simulink model "ExampleStorageDoubleTempAssignment"  (R2016a)
settings: Solver=VariableStepAuto  StartTime=0.0  StopTime=3600*10  RelTol=1e-3
settings Model: Creator=chiavazzo  LastModifiedBy=chiavazzo

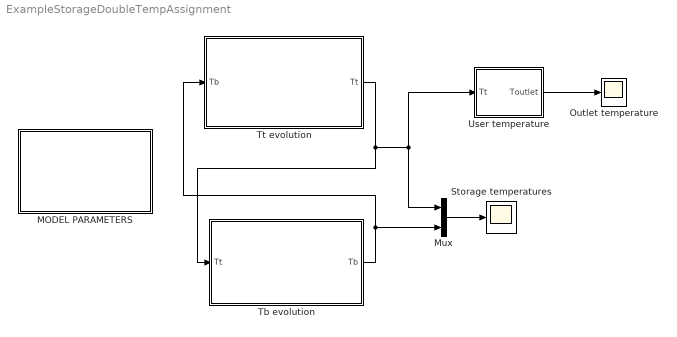
== system ExampleStorageDoubleTempAssignment ==
  " Outlet temperature" : Scope
  MODEL PARAMETERS : Subsystem
  Mux : Mux  Inputs=2
  Storage temperatures : Scope
  Tb evolution : Subsystem
  Tt evolution : Subsystem
  User temperature : Subsystem
  wires:
  Tt evolution/1(Tt) -> User temperature/1(Tt), Mux/1, Tb evolution/1(Tt)
  Tb evolution/1(Tb) -> Tt evolution/1(Tb), Mux/2
  Mux/1 -> Storage temperatures/1
  User temperature/1(Toutlet) -> " Outlet temperature"/1

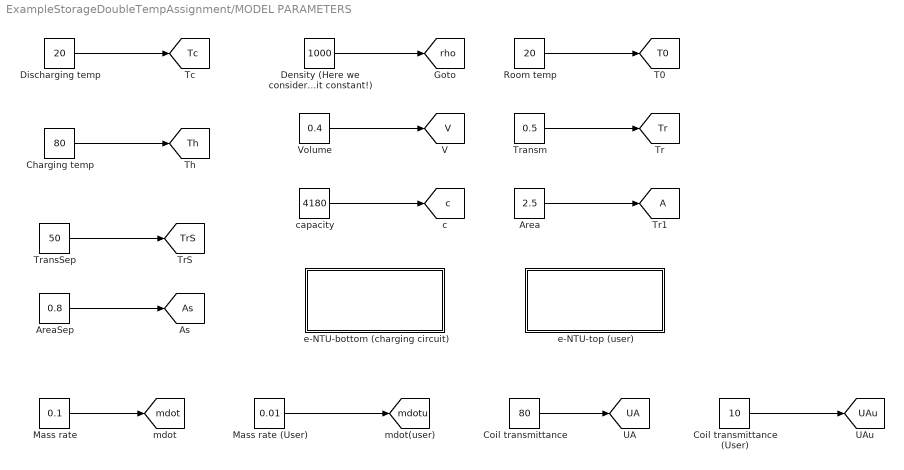
== system ExampleStorageDoubleTempAssignment/MODEL PARAMETERS ==
  Area : Constant  Value=2.5
  AreaSep : Constant  Value=0.8
  Charging temp : Constant  Value=80
  Coil transmittance : Constant  Value=80
  Coil transmittance (User) : Constant  Value=10
  Density (Here we consider it constant!) : Constant  Value=1000
  Discharging temp : Constant  Value=20
  Mass rate : Constant  Value=0.1
  Mass rate (User) : Constant  Value=0.01
  Room temp : Constant  Value=20
  TransSep : Constant  Value=50
  Transm : Constant  Value=0.5
  Volume : Constant  Value=0.4
  capacity : Constant  Value=4180
  e-NTU-bottom (charging circuit) : Subsystem
  e-NTU-top (user) : Subsystem
  tag scope: A=global, As=global, T0=global, Tc=global, Th=global, Tr=global, TrS=global, UA=global, UAu=global, V=global, c=global, mdot=global, mdotu=global, rho=global
  wires:
  Volume/1 -> [V]
  Coil transmittance/1 -> [UA]
  Mass rate/1 -> [mdot]
  capacity/1 -> [c]
  Area/1 -> [A]
  Room temp/1 -> [T0]
  Density (Here we consider it constant!)/1 -> [rho]
  Transm/1 -> [Tr]
  Charging temp/1 -> [Th]
  TransSep/1 -> [TrS]
  AreaSep/1 -> [As]
  Discharging temp/1 -> [Tc]
  Coil transmittance (User)/1 -> [UAu]
  Mass rate (User)/1 -> [mdotu]

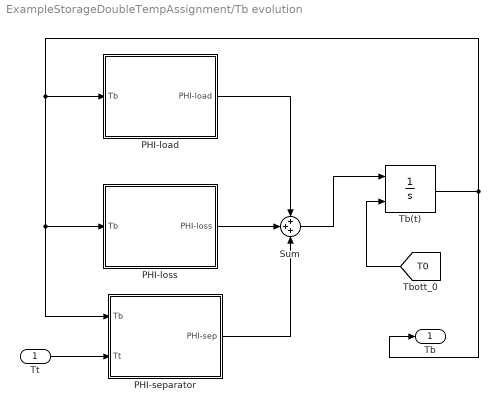
== system ExampleStorageDoubleTempAssignment/Tb evolution ==
  Tt : Inport
  PHI-load : Subsystem
  PHI-loss : Subsystem
  PHI-separator : Subsystem
  Sum : Sum  Inputs=+++
  Tb(t) : Integrator  InitialConditionSource=external
  Tb : Outport
  wires:
  PHI-loss/1(PHI-loss) -> Sum/2
  Sum/1 -> Tb(t)/1
  PHI-load/1(PHI-load) -> Sum/1
  [T0] -> Tb(t)/2
  Tb(t)/1 -> Tb/1, PHI-separator/1(Tb), PHI-loss/1(Tb), PHI-load/1(Tb)
  PHI-separator/1(PHI-sep) -> Sum/3
  Tt/1 -> PHI-separator/2(Tt)

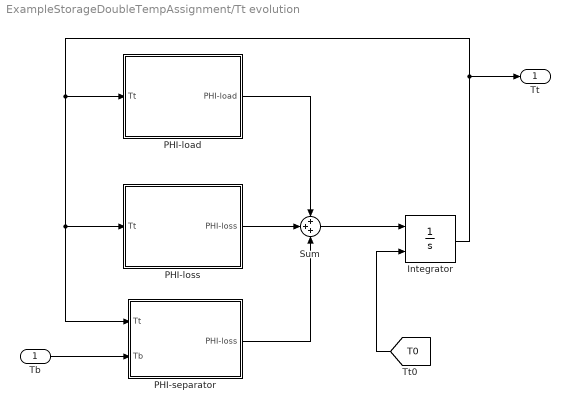
== system ExampleStorageDoubleTempAssignment/Tt evolution ==
  Tb : Inport
  Integrator : Integrator  InitialConditionSource=external
  PHI-load : Subsystem
  PHI-loss : Subsystem
  PHI-separator : Subsystem
  Sum : Sum  Inputs=+++
  Tt : Outport
  wires:
  PHI-loss/1(PHI-loss) -> Sum/2
  Sum/1 -> Integrator/1
  PHI-load/1(PHI-load) -> Sum/1
  [T0] -> Integrator/2
  Integrator/1 -> Tt/1, PHI-separator/1(Tt), PHI-loss/1(Tt), PHI-load/1(Tt)
  PHI-separator/1(PHI-loss) -> Sum/3
  Tb/1 -> PHI-separator/2(Tb)

== system ExampleStorageDoubleTempAssignment/User temperature ==
  Tt : Inport
  Product : Product
  Sum : Sum  Inputs=|+-
  Sum1 : Sum  Inputs=|++
  Toutlet : Outport
  wires:
  [epsu] -> Product/1
  Sum1/1 -> Toutlet/1
  Sum/1 -> Product/2
  [Tc] -> Sum/2
  [Tc] -> Sum1/1
  Product/1 -> Sum1/2
  Tt/1 -> Sum/1

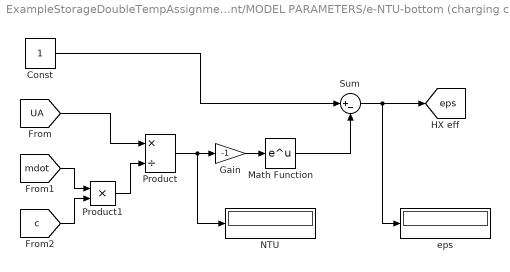
== system ExampleStorageDoubleTempAssignment/MODEL PARAMETERS/e-NTU-bottom (charging circuit) ==
  Const : Constant
  Gain : Gain  Gain=-1
  Math Function : Math  SaturateOnIntegerOverflow=on
  NTU : Display
  Product : Product  Inputs=*/
  Product1 : Product  Inputs=**
  Sum : Sum  Inputs=|+-
  eps : Display
  tag scope: eps=global
  wires:
  [mdot] -> Product1/1
  Product/1 -> NTU/1, Gain/1
  Product1/1 -> Product/2
  [UA] -> Product/1
  Sum/1 -> eps/1, [eps]
  Const/1 -> Sum/1
  Math Function/1 -> Sum/2
  Gain/1 -> Math Function/1
  [c] -> Product1/2

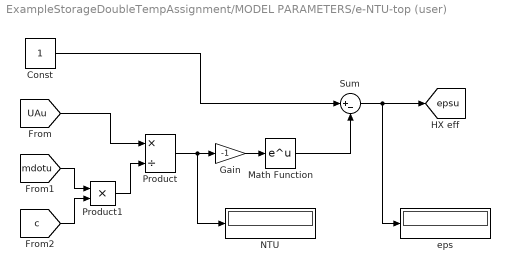
== system ExampleStorageDoubleTempAssignment/MODEL PARAMETERS/e-NTU-top (user) ==
  Const : Constant
  Gain : Gain  Gain=-1
  Math Function : Math  SaturateOnIntegerOverflow=on
  NTU : Display
  Product : Product  Inputs=*/
  Product1 : Product  Inputs=**
  Sum : Sum  Inputs=|+-
  eps : Display
  tag scope: epsu=global
  wires:
  [mdotu] -> Product1/1
  Product/1 -> NTU/1, Gain/1
  Product1/1 -> Product/2
  [UAu] -> Product/1
  Sum/1 -> eps/1, [epsu]
  Const/1 -> Sum/1
  Math Function/1 -> Sum/2
  Gain/1 -> Math Function/1
  [c] -> Product1/2

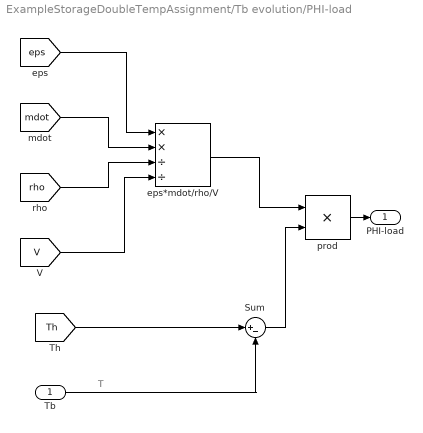
== system ExampleStorageDoubleTempAssignment/Tb evolution/PHI-load ==
  note: T
  Tb : Inport
  Sum : Sum  Inputs=|+-
  eps*mdot/rho/V : Product  Inputs=**//
  prod : Product  Inputs=**
  PHI-load : Outport
  wires:
  eps*mdot/rho/V/1 -> prod/1
  [V] -> eps*mdot/rho/V/4
  [mdot] -> eps*mdot/rho/V/2
  Sum/1 -> prod/2
  [rho] -> eps*mdot/rho/V/3
  [Th] -> Sum/1
  Tb/1 -> Sum/2
  prod/1 -> PHI-load/1
  [eps] -> eps*mdot/rho/V/1

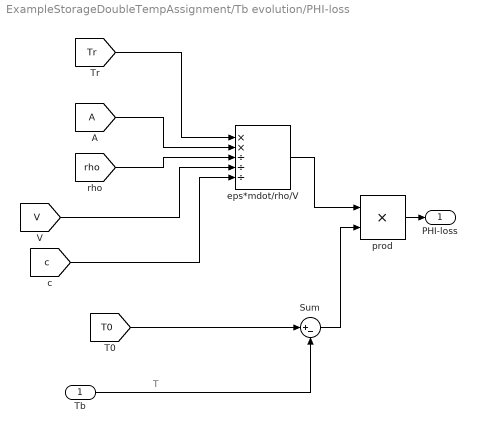
== system ExampleStorageDoubleTempAssignment/Tb evolution/PHI-loss ==
  note: T
  Tb : Inport
  Sum : Sum  Inputs=|+-
  eps*mdot/rho/V : Product  Inputs=**///
  prod : Product  Inputs=**
  PHI-loss : Outport
  wires:
  eps*mdot/rho/V/1 -> prod/1
  [V] -> eps*mdot/rho/V/4
  [A] -> eps*mdot/rho/V/2
  Sum/1 -> prod/2
  [rho] -> eps*mdot/rho/V/3
  [T0] -> Sum/1
  Tb/1 -> Sum/2
  prod/1 -> PHI-loss/1
  [Tr] -> eps*mdot/rho/V/1
  [c] -> eps*mdot/rho/V/5

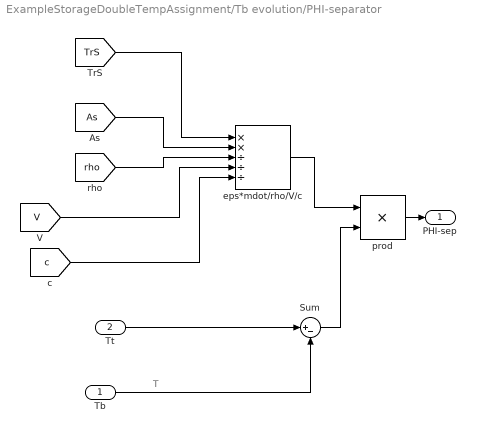
== system ExampleStorageDoubleTempAssignment/Tb evolution/PHI-separator ==
  note: T
  Tb : Inport
  Tt : Inport  Port=2
  Sum : Sum  Inputs=|+-
  eps*mdot/rho/V/c : Product  Inputs=**///
  prod : Product  Inputs=**
  PHI-sep : Outport
  wires:
  eps*mdot/rho/V/c/1 -> prod/1
  [V] -> eps*mdot/rho/V/c/4
  [As] -> eps*mdot/rho/V/c/2
  Sum/1 -> prod/2
  [rho] -> eps*mdot/rho/V/c/3
  Tt/1 -> Sum/1
  Tb/1 -> Sum/2
  prod/1 -> PHI-sep/1
  [TrS] -> eps*mdot/rho/V/c/1
  [c] -> eps*mdot/rho/V/c/5

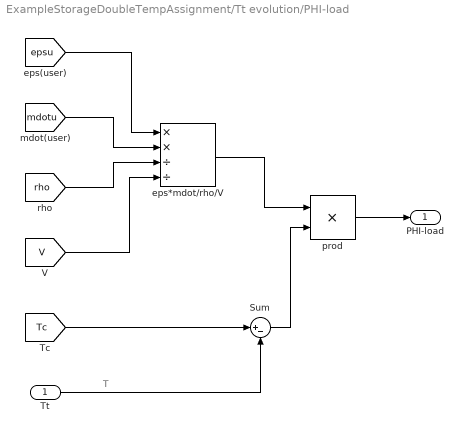
== system ExampleStorageDoubleTempAssignment/Tt evolution/PHI-load ==
  note: T
  Tt : Inport
  Sum : Sum  Inputs=|+-
  eps*mdot/rho/V : Product  Inputs=**//
  prod : Product  Inputs=**
  PHI-load : Outport
  wires:
  eps*mdot/rho/V/1 -> prod/1
  [V] -> eps*mdot/rho/V/4
  [mdotu] -> eps*mdot/rho/V/2
  Sum/1 -> prod/2
  [rho] -> eps*mdot/rho/V/3
  [Tc] -> Sum/1
  Tt/1 -> Sum/2
  prod/1 -> PHI-load/1
  [epsu] -> eps*mdot/rho/V/1

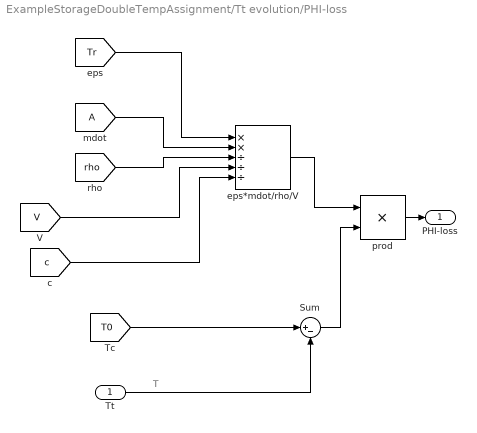
== system ExampleStorageDoubleTempAssignment/Tt evolution/PHI-loss ==
  note: T
  Tt : Inport
  Sum : Sum  Inputs=|+-
  eps*mdot/rho/V : Product  Inputs=**///
  prod : Product  Inputs=**
  PHI-loss : Outport
  wires:
  eps*mdot/rho/V/1 -> prod/1
  [V] -> eps*mdot/rho/V/4
  [A] -> eps*mdot/rho/V/2
  Sum/1 -> prod/2
  [rho] -> eps*mdot/rho/V/3
  [T0] -> Sum/1
  Tt/1 -> Sum/2
  prod/1 -> PHI-loss/1
  [Tr] -> eps*mdot/rho/V/1
  [c] -> eps*mdot/rho/V/5

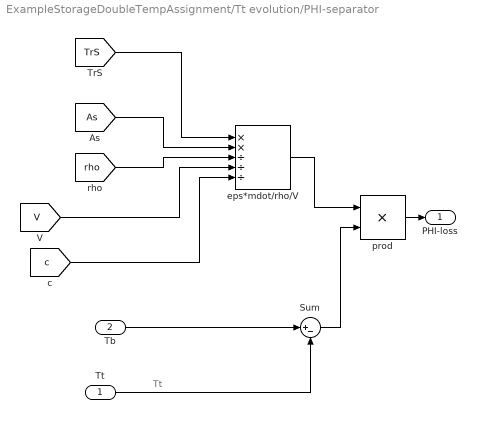
== system ExampleStorageDoubleTempAssignment/Tt evolution/PHI-separator ==
  note: Tt
  Tt : Inport
  Tb : Inport  Port=2
  Sum : Sum  Inputs=|+-
  eps*mdot/rho/V : Product  Inputs=**///
  prod : Product  Inputs=**
  PHI-loss : Outport
  wires:
  eps*mdot/rho/V/1 -> prod/1
  [V] -> eps*mdot/rho/V/4
  [As] -> eps*mdot/rho/V/2
  Sum/1 -> prod/2
  [rho] -> eps*mdot/rho/V/3
  Tb/1 -> Sum/1
  Tt/1 -> Sum/2
  prod/1 -> PHI-loss/1
  [TrS] -> eps*mdot/rho/V/1
  [c] -> eps*mdot/rho/V/5
